simulink model "Shubert"  (R2019a)
settings: Solver=FixedStepAuto  StartTime=0.0  StopTime=size(InputValues_20200610T231852540,1) - 1  FixedStep=1  RelTol=1e-3
model workspace (MAT data in the model file):
  InputValues_20200610T231852540 = [0 0.0245361328125 0.049072265625 0.0736083984375 0.09814453125 0.122680664062 0.147216796875 0.171752929688 0.1962890625 0.220825195312 0.245361328125 0.269897460938 ... (257 elements, 257x1)]
libraries: simulink x1
settings Model: OrderedModelArguments=off  Creator=letras  LastModifiedBy=letras
settings DebuggingCC: IntegerOverflowMsg=none  ParameterOverflowMsg=none  ParameterPrecisionLossMsg=none  IntegerSaturationMsg=none

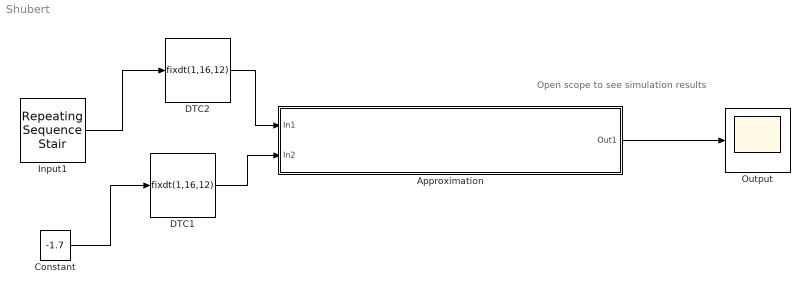
== system Shubert ==
  note: Open scope to see simulation results
  Approximation : Subsystem  Description=This block was created using function approximation.
  Constant : Constant  Value=-1.7
  DTC1 : DataTypeConversion  OutDataTypeStr=fixdt(1,16,12)  RndMeth=Nearest
  DTC2 : DataTypeConversion  OutDataTypeStr=fixdt(1,16,12)  RndMeth=Nearest
  Input1 : simulink/Sources/Repeating Sequence Stair  OutValues=[-5 -4 -3 -2 -1 0 1 2 3 4 5]  tsamp=-1  OutMin=[]  OutMax=[]  OutDataTypeStr=double  OutputDataTypeScalingMode=double  OutDataType=fixdt(0,8)  ConRadixGroup=Best Precision: Vector-wise  OutScaling=2^-12
  Output : Scope
  wires:
  Input1/1 -> DTC2/1
  Approximation/1(Out1) -> Output/1
  DTC1/1 -> Approximation/2(In2)
  DTC2/1 -> Approximation/1(In1)
  Constant/1 -> DTC1/1

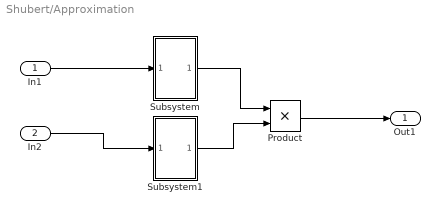
== system Shubert/Approximation ==
  In1 : Inport
  In2 : Inport  Port=2
  Product : Product
  Subsystem : Subsystem
  Subsystem1 : Subsystem
  Out1 : Outport
  wires:
  In1/1 -> Subsystem/1(In1)
  Subsystem/1(Out1) -> Product/1
  Product/1 -> Out1/1
  Subsystem1/1(Out1) -> Product/2
  In2/1 -> Subsystem1/1(In1)

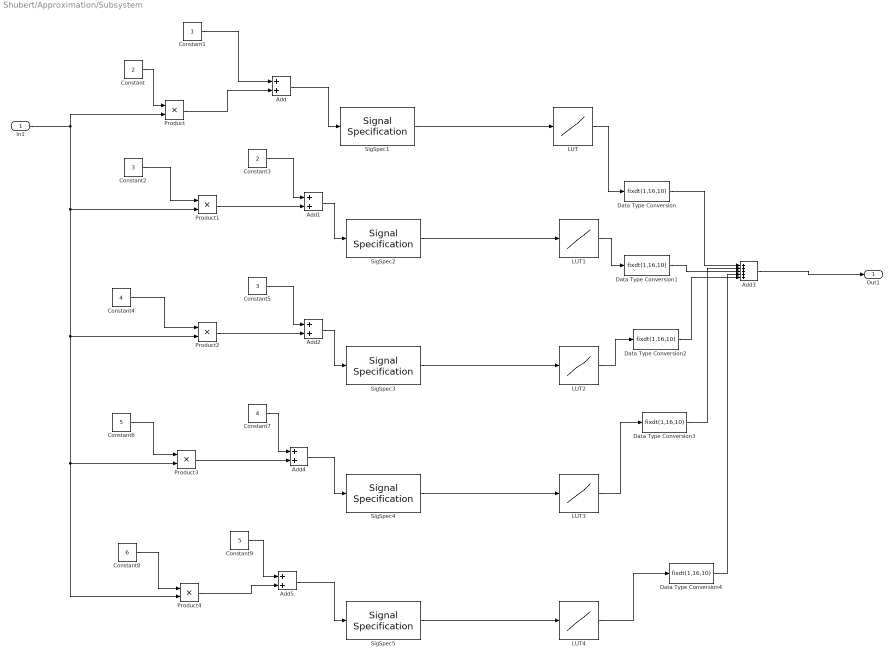
== system Shubert/Approximation/Subsystem ==
  In1 : Inport
  Add{,1..2,4..5} (5 alike) : Sum  AccumDataTypeStr=fixdt(1,16,9)
  Add3 : Sum  Inputs=+++++  AccumDataTypeStr=fixdt(1,16,10)
  Constant : Constant  Value=2  OutDataTypeStr=fixdt(0,16,13)
  Constant1 : Constant  OutDataTypeStr=fixdt(0,16,14)
  Constant2 : Constant  Value=3  OutDataTypeStr=fixdt(0,16,13)
  Constant3 : Constant  Value=2  OutDataTypeStr=fixdt(0,16,13)
  Constant4 : Constant  Value=4  OutDataTypeStr=fixdt(0,16,13)
  Constant5 : Constant  Value=3  OutDataTypeStr=fixdt(0,16,13)
  Constant6 : Constant  Value=5  OutDataTypeStr=fixdt(0,16,13)
  Constant7 : Constant  Value=4  OutDataTypeStr=fixdt(0,16,13)
  Constant8 : Constant  Value=6  OutDataTypeStr=fixdt(0,16,13)
  Constant9 : Constant  Value=5  OutDataTypeStr=fixdt(0,16,13)
  Data Type Conversion{,1..4} (5 alike) : DataTypeConversion  OutDataTypeStr=fixdt(1,16,10)
  LUT{,1..4} (5 alike) : Lookup_n-D  NumberOfTableDimensions=1  LookupTableObject=FunctionApproximation_LUTObject_20210714T214041645  BreakpointsSpecification=Even spacing  BreakpointsForDimension3=[5, 7]  BreakpointsForDimension1FirstPoint=-25  BreakpointsForDimension1DataTypeStr=numerictype(1,16,9)  IndexSearchMethod=Evenly spaced points  Table=[0.9912109375 0.4241943359375 -0.5328369140625 -0.99993896484375 -0.5477294921875 0.4080810546875 0.98870849609375 0.66033935546875 -0.275146484375 -0.9576416015625 -0.75970458984375 0.13671875 0.907470703125 0.8438720703125 0.00445556640625 -0.83905029296875 -0.9111328125 -0.1455078125 0.75390625 0.96014404296875 0.28369140625 -0.65362548828125 -0.989990234375 -0.4161376953125 0.540283203125 1 0.540283203125 -0.4161376953125 -0.989990234375 -0.65362548828125 0.28369140625 0.96014404296875 0.75390625 -0.1455078125 -0.9111328125 -0.83905029296875 0.00445556640625 0.8438720703125 0.907470703125 0.13671875 -0.75970458984375 -0.9576416015625 -0.275146484375 0.66033935546875 0.98870849609375 0.4080810546875 -0.5477294921875 -0.99993896484375 -0.5328369140625 0.4241943359375 0.9912109375 0.64691162109375 -0.2921142578125 -0.96258544921875 -0.748046875 0.15423583984375 0.91473388671875 0.834228515625 -0.0133056640625 -0.84857177734375 -0.9036865234375]  TableDataTypeStr=numerictype(1,16,14)  ExtrapMethod=Clip  UseLastTableValue=on  InternalRulePriority=Speed  OutDataTypeStr=numerictype(1,16,14)  RndMeth=Simplest
  Product{,1..4} (5 alike) : Product  OutDataTypeStr=fixdt(1,16,9)
  SigSpec{1..5} (5 alike) : SignalSpecification  OutMin=0  OutMax=6.283203125  OutDataTypeStr=numerictype(1,16,9)
  Out1 : Outport
  wires:
  SigSpec2/1 -> LUT1/1
  Constant1/1 -> Add/1
  Constant3/1 -> Add1/1
  Constant/1 -> Product/1
  Constant4/1 -> Product2/1
  Add1/1 -> SigSpec2/1
  Constant6/1 -> Product3/1
  Product3/1 -> Add4/2
  Product1/1 -> Add1/2
  Constant2/1 -> Product1/1
  Constant9/1 -> Add5/1
  Add3/1 -> Out1/1
  SigSpec1/1 -> LUT/1
  Constant5/1 -> Add2/1
  Constant8/1 -> Product4/1
  Add4/1 -> SigSpec4/1
  Add2/1 -> SigSpec3/1
  In1/1 -> Product/2, Product1/2, Product4/2, Product3/2, Product2/2
  Add5/1 -> SigSpec5/1
  Product4/1 -> Add5/2
  Product/1 -> Add/2
  Product2/1 -> Add2/2
  Add/1 -> SigSpec1/1
  SigSpec5/1 -> LUT4/1
  SigSpec3/1 -> LUT2/1
  Constant7/1 -> Add4/1
  SigSpec4/1 -> LUT3/1
  LUT/1 -> Data Type Conversion/1
  Data Type Conversion/1 -> Add3/1
  LUT1/1 -> Data Type Conversion1/1
  Data Type Conversion1/1 -> Add3/3
  LUT2/1 -> Data Type Conversion2/1
  Data Type Conversion2/1 -> Add3/5
  LUT3/1 -> Data Type Conversion3/1
  Data Type Conversion3/1 -> Add3/2
  LUT4/1 -> Data Type Conversion4/1
  Data Type Conversion4/1 -> Add3/4

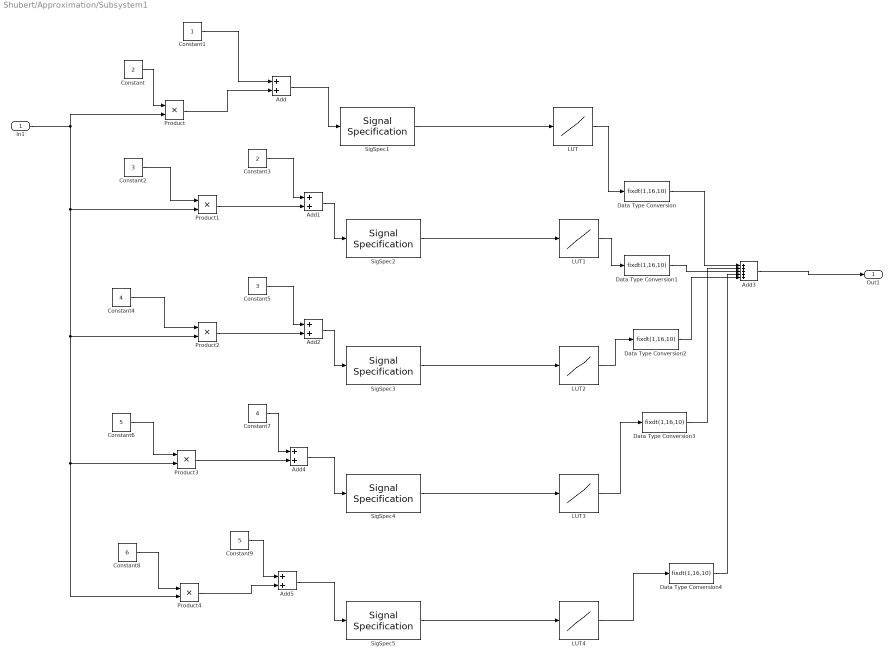
== system Shubert/Approximation/Subsystem1 ==
  In1 : Inport
  Add{,1..2,4..5} (5 alike) : Sum  AccumDataTypeStr=fixdt(1,16,9)
  Add3 : Sum  Inputs=+++++  AccumDataTypeStr=fixdt(1,16,10)
  Constant : Constant  Value=2  OutDataTypeStr=fixdt(0,16,13)
  Constant1 : Constant  OutDataTypeStr=fixdt(0,16,14)
  Constant2 : Constant  Value=3  OutDataTypeStr=fixdt(0,16,13)
  Constant3 : Constant  Value=2  OutDataTypeStr=fixdt(0,16,13)
  Constant4 : Constant  Value=4  OutDataTypeStr=fixdt(0,16,13)
  Constant5 : Constant  Value=3  OutDataTypeStr=fixdt(0,16,13)
  Constant6 : Constant  Value=5  OutDataTypeStr=fixdt(0,16,13)
  Constant7 : Constant  Value=4  OutDataTypeStr=fixdt(0,16,13)
  Constant8 : Constant  Value=6  OutDataTypeStr=fixdt(0,16,13)
  Constant9 : Constant  Value=5  OutDataTypeStr=fixdt(0,16,13)
  Data Type Conversion{,1..4} (5 alike) : DataTypeConversion  OutDataTypeStr=fixdt(1,16,10)
  LUT{,1..4} (5 alike) : Lookup_n-D  NumberOfTableDimensions=1  LookupTableObject=FunctionApproximation_LUTObject_20210714T214041645  BreakpointsSpecification=Even spacing  BreakpointsForDimension3=[5, 7]  BreakpointsForDimension1FirstPoint=-25  BreakpointsForDimension1DataTypeStr=numerictype(1,16,9)  IndexSearchMethod=Evenly spaced points  Table=[0.9912109375 0.4241943359375 -0.5328369140625 -0.99993896484375 -0.5477294921875 0.4080810546875 0.98870849609375 0.66033935546875 -0.275146484375 -0.9576416015625 -0.75970458984375 0.13671875 0.907470703125 0.8438720703125 0.00445556640625 -0.83905029296875 -0.9111328125 -0.1455078125 0.75390625 0.96014404296875 0.28369140625 -0.65362548828125 -0.989990234375 -0.4161376953125 0.540283203125 1 0.540283203125 -0.4161376953125 -0.989990234375 -0.65362548828125 0.28369140625 0.96014404296875 0.75390625 -0.1455078125 -0.9111328125 -0.83905029296875 0.00445556640625 0.8438720703125 0.907470703125 0.13671875 -0.75970458984375 -0.9576416015625 -0.275146484375 0.66033935546875 0.98870849609375 0.4080810546875 -0.5477294921875 -0.99993896484375 -0.5328369140625 0.4241943359375 0.9912109375 0.64691162109375 -0.2921142578125 -0.96258544921875 -0.748046875 0.15423583984375 0.91473388671875 0.834228515625 -0.0133056640625 -0.84857177734375 -0.9036865234375]  TableDataTypeStr=numerictype(1,16,14)  ExtrapMethod=Clip  UseLastTableValue=on  InternalRulePriority=Speed  OutDataTypeStr=numerictype(1,16,14)  RndMeth=Simplest
  Product{,1..4} (5 alike) : Product  OutDataTypeStr=fixdt(1,16,9)
  SigSpec{1..5} (5 alike) : SignalSpecification  OutMin=0  OutMax=6.283203125  OutDataTypeStr=numerictype(1,16,9)
  Out1 : Outport
  wires:
  SigSpec2/1 -> LUT1/1
  Constant1/1 -> Add/1
  Constant3/1 -> Add1/1
  Constant/1 -> Product/1
  Constant4/1 -> Product2/1
  Add1/1 -> SigSpec2/1
  Constant6/1 -> Product3/1
  Product3/1 -> Add4/2
  Product1/1 -> Add1/2
  Constant2/1 -> Product1/1
  Constant9/1 -> Add5/1
  Add3/1 -> Out1/1
  SigSpec1/1 -> LUT/1
  Constant5/1 -> Add2/1
  Constant8/1 -> Product4/1
  Add4/1 -> SigSpec4/1
  Add2/1 -> SigSpec3/1
  In1/1 -> Product/2, Product1/2, Product4/2, Product3/2, Product2/2
  Add5/1 -> SigSpec5/1
  Product4/1 -> Add5/2
  Product/1 -> Add/2
  Product2/1 -> Add2/2
  Add/1 -> SigSpec1/1
  SigSpec5/1 -> LUT4/1
  SigSpec3/1 -> LUT2/1
  Constant7/1 -> Add4/1
  SigSpec4/1 -> LUT3/1
  LUT/1 -> Data Type Conversion/1
  Data Type Conversion/1 -> Add3/1
  LUT1/1 -> Data Type Conversion1/1
  Data Type Conversion1/1 -> Add3/3
  LUT2/1 -> Data Type Conversion2/1
  Data Type Conversion2/1 -> Add3/5
  LUT3/1 -> Data Type Conversion3/1
  Data Type Conversion3/1 -> Add3/2
  LUT4/1 -> Data Type Conversion4/1
  Data Type Conversion4/1 -> Add3/4
